simulink model "quadrotor_formationDEM_Fire_singleWPNAV"  (R2021a)
settings: Solver=VariableStepAuto  StartTime=0.0  StopTime=22000  RelTol=1e-3
values from neighbouring files (symbols this model uses):
  centroidi2 = cen_input'    [adj_cen.m]
  initialCondition = [x0 vx0 y0 vy0 z0 vz0 phi0 p0 theta0 q0 psi0 r0]    [variables.m]
  initialCondition2 = [x02 vx0 y02 vy0 z2 vz0 phi0 p0 theta0 q0 psi0 r0]    [variables.m]
  initialCondition3 = [x03 vx0 y03 vy0 z3 vz0 phi0 p0 theta0 q0 psi0 r0]    [variables.m]
  numero_wp = col    [adj_cen.m]
undefined symbols (not defined in the file or in its folder): tensore
settings Model: Creator=fiori  LastModifiedBy=fiori
settings SolverCC: AlgebraicLoopSolver=TrustRegion
settings DebuggingCC: SFMachineParentedDataDiag=warning

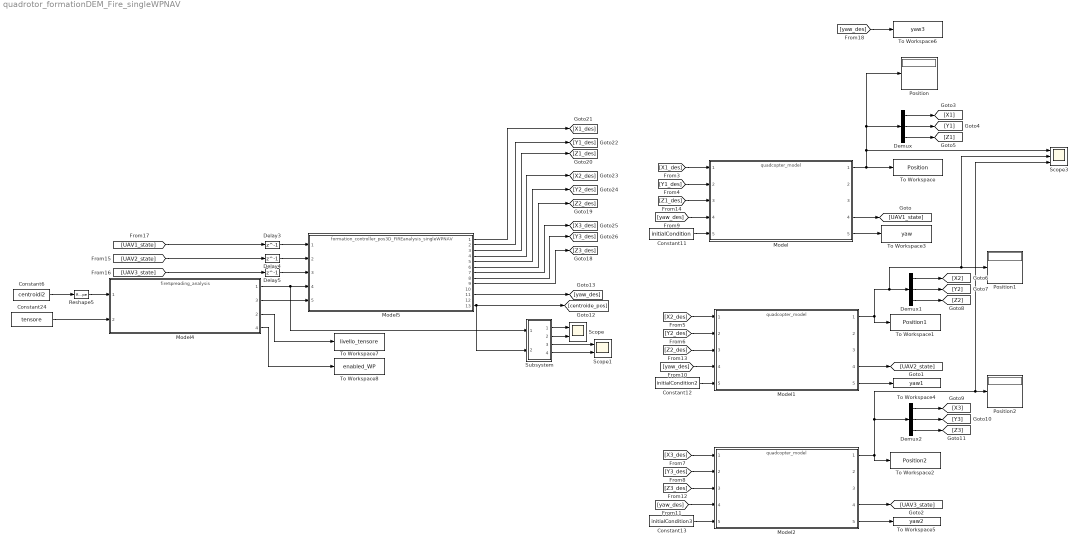
== system quadrotor_formationDEM_Fire_singleWPNAV ==
  Constant11 : Constant  Value=initialCondition
  Constant12 : Constant  Value=initialCondition2
  Constant13 : Constant  Value=initialCondition3
  Constant24 : Constant  Value=tensore
  Constant6 : Constant  Value=centroidi2
  Delay3 : Delay  DelayLength=1  InitialCondition=0  SampleTime=0.1
  Delay4 : Delay  DelayLength=1  InitialCondition=0  SampleTime=0.1
  Delay5 : Delay  DelayLength=1  InitialCondition=0  SampleTime=0.1
  Demux : Demux  Outputs=3
  Demux1 : Demux  Outputs=3
  Demux2 : Demux  Outputs=3
  Model : ModelReference  ModelNameDialog=quadcopter_model.slx  SimulationMode=Normal  ModelReferenceVersion=3.0
  Model1 : ModelReference  ModelNameDialog=quadcopter_model.slx  SimulationMode=Normal  ModelReferenceVersion=3.0
  Model2 : ModelReference  ModelNameDialog=quadcopter_model.slx  SimulationMode=Normal  ModelReferenceVersion=3.0
  Model4 : ModelReference  ModelNameDialog=fireSpreading_analysis.slx  SimulationMode=Normal  ModelReferenceVersion=2.12
      settings: PortSchema="{\"entries\":[{\"content\":{\"sides\":[{\"content\":{\"connectorIds\":[\"In1\",\"In2\"]},\"type\":\"ConnectorPlacement.EquallySpacedRectSide\",\"uuid\":\"638b7215-e002-4d3c-b29e-ef26dedc51b1\"},{\"content\":{\"connectorIds\":[\"Out1\",\"Out3\",\"Out2\",\"Out4\"],\"side\":\"RIGHT\"},\"type\":\"ConnectorPlacement.EquallySpacedRectSide\",\"uuid\":\"32a720be-6519-420b-ab39-cb798e793d5c\"},{\"content\":{\"connectorIds\":[],\"side\":\"TOP\"},\"type\":\"ConnectorPlacement.EquallySpacedRectSide\",\"uuid\":\"5662e1bc-995f-46f6-9c84-3a19c7d97029\"}]},\"type\":\"ConnectorPlacement.EquallySpacedConnector\",\"uuid\":\"03419422-6d30-4f4d-94e5-e3ebd9093609\"}],\"packageUris\":[\"http://schema.mathworks.com/mf0/Connector/R2020b\"],\"version\":\"1.0\"}"
  Model5 : ModelReference  ModelNameDialog=formation_controller_pos3D_FIREanalysis_singleWPNAV.slx  SimulationMode=Normal  ModelReferenceVersion=2.2
  Position : Display
  Position1 : Display
  Position2 : Display
  Reshape5 : Reshape  OutputDimensionality=Customize  OutputDimensions=[3,numero_wp]
  Scope : Scope  NumInputPorts=2
  Scope1 : Scope  NumInputPorts=2
  Scope3 : Scope  NumInputPorts=3
  Subsystem : Subsystem
  To Workspace : ToWorkspace  VariableName=Position  SaveFormat=Structure With Time  SampleTime=-1
  To Workspace1 : ToWorkspace  VariableName=Position1  SaveFormat=Structure With Time  SampleTime=-1
  To Workspace2 : ToWorkspace  VariableName=Position2  SaveFormat=Structure With Time  SampleTime=-1
  To Workspace3 : ToWorkspace  VariableName=yaw  SaveFormat=Structure With Time  SampleTime=-1
  To Workspace4 : ToWorkspace  VariableName=yaw1  SaveFormat=Structure With Time  SampleTime=-1
  To Workspace5 : ToWorkspace  VariableName=yaw2  SaveFormat=Structure With Time  SampleTime=-1
  To Workspace6 : ToWorkspace  VariableName=yaw3  SaveFormat=Structure With Time  SampleTime=-1
  To Workspace7 : ToWorkspace  VariableName=livello_tensore  SaveFormat=Structure With Time  SampleTime=-1
  To Workspace8 : ToWorkspace  VariableName=enabled_WP  SaveFormat=Structure With Time  SampleTime=-1
  wires:
  Model/1 -> To Workspace/1, Position/1, Demux/1, Scope3/1
  Model/4 -> [UAV1_state]
  Model1/4 -> [UAV2_state]
  Model2/4 -> [UAV3_state]
  Constant11/1 -> Model/5
  Constant12/1 -> Model1/5
  Constant13/1 -> Model2/5
  Demux/1 -> [X1]
  Demux/2 -> [Y1]
  Demux/3 -> [Z1]
  Demux1/1 -> [X2]
  Model1/1 -> To Workspace1/1, Scope3/2, Position1/1, Demux1/1
  Demux1/3 -> [Z2]
  Demux1/2 -> [Y2]
  Demux2/1 -> [X3]
  Model2/1 -> To Workspace2/1, Scope3/3, Position2/1, Demux2/1
  Demux2/3 -> [Z3]
  Demux2/2 -> [Y3]
  [Y1_des] -> Model/2
  [X1_des] -> Model/1
  [Y2_des] -> Model1/2
  [X2_des] -> Model1/1
  [Y3_des] -> Model2/2
  [X3_des] -> Model2/1
  Model5/9 -> [Z3_des]
  Model5/6 -> [Z2_des]
  Model5/3 -> [Z1_des]
  [UAV2_state] -> Delay4/1
  [UAV3_state] -> Delay5/1
  [UAV1_state] -> Delay3/1
  Model5/5 -> [Y2_des]
  Model5/8 -> [Y3_des]
  Model5/4 -> [X2_des]
  Model5/2 -> [Y1_des]
  Model5/7 -> [X3_des]
  Model5/1 -> [X1_des]
  Model/5 -> To Workspace3/1
  Model1/5 -> To Workspace4/1
  Model2/5 -> To Workspace5/1
  [Z1_des] -> Model/3
  [Z2_des] -> Model1/3
  [Z3_des] -> Model2/3
  Model5/11 -> [yaw_des]
  [yaw_des] -> Model/4
  [yaw_des] -> Model1/4
  [yaw_des] -> Model2/4
  [yaw_des] -> To Workspace6/1
  Constant6/1 -> Reshape5/1
  Reshape5/1 -> Model4/1
  Constant24/1 -> Model4/2
  Model4/1 -> Subsystem/1(In1), Model5/4
  Model4/3 -> Model5/5
  Model4/2 -> To Workspace7/1
  Model4/4 -> To Workspace8/1
  Model5/13 -> Subsystem/2(In2), [centroide_pos]
  Delay3/1 -> Model5/1
  Delay4/1 -> Model5/2
  Delay5/1 -> Model5/3
  Subsystem/1(Out1) -> Scope/1
  Subsystem/2(Out2) -> Scope/2
  Subsystem/3(Out3) -> Scope1/1
  Subsystem/4(Out4) -> Scope1/2

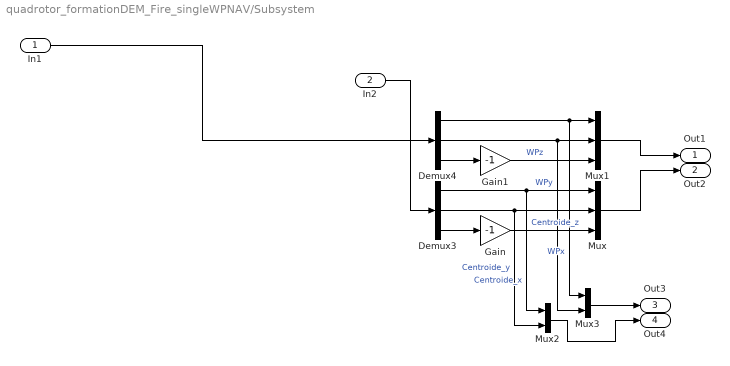
== system quadrotor_formationDEM_Fire_singleWPNAV/Subsystem ==
  In1 : Inport
  In2 : Inport  Port=2
  Demux3 : Demux  Outputs=3
  Demux4 : Demux  Outputs=3
  Gain : Gain  Gain=-1
  Gain1 : Gain  Gain=-1
  Mux : Mux  Inputs=3
  Mux1 : Mux  Inputs=3
  Mux2 : Mux  Inputs=2
  Mux3 : Mux  Inputs=2
  Out1 : Outport
  Out2 : Outport  Port=2
  Out3 : Outport  Port=3
  Out4 : Outport  Port=4
  wires:
  Demux3/3 -> Gain/1
  Demux3/2 -> Mux2/2, Mux/2  "Centroide_y"
  Gain1/1 -> Mux1/3  "WPz"
  Demux3/1 -> Mux2/1, Mux/1  "Centroide_x"
  Demux4/2 -> Mux1/2, Mux3/2  "WPy"
  Demux4/3 -> Gain1/1
  Mux2/1 -> Out4/1
  Gain/1 -> Mux/3  "Centroide_z"
  Demux4/1 -> Mux3/1, Mux1/1  "WPx"
  In2/1 -> Demux3/1
  Mux/1 -> Out2/1
  Mux1/1 -> Out1/1
  Mux3/1 -> Out3/1
  In1/1 -> Demux4/1
